simulink model "Modeling"  (R2022b)
settings: Solver=VariableStepAuto  StartTime=0.0  StopTime=2.5  RelTol=1e-3
values from neighbouring files (symbols this model uses):
  b_m = 0.002953    [Modeling_constants.m]
  g = 9.81    [Modeling_constants.m]
  j_m = 0.0221    [Modeling_constants.m]
  j_w = 0.01581762    [Modeling_constants.m]
  K_b = 0.25    [Modeling_constants.m]
  K_m = 0.516    [Modeling_constants.m]
  L_a = 0.0281    [Modeling_constants.m]
  M = 1 / 2    (= 0.5)    [Modeling_constants.m]
  m = 0.5    [Modeling_constants.m]
  r = 0.0325    [Modeling_constants.m]
  R_a = 2.581    [Modeling_constants.m]
  V_i = 450    [Modeling_constants.m]
libraries: slpidlib x2
settings Model: Creator=a7mad  LastModifiedBy=a7mad

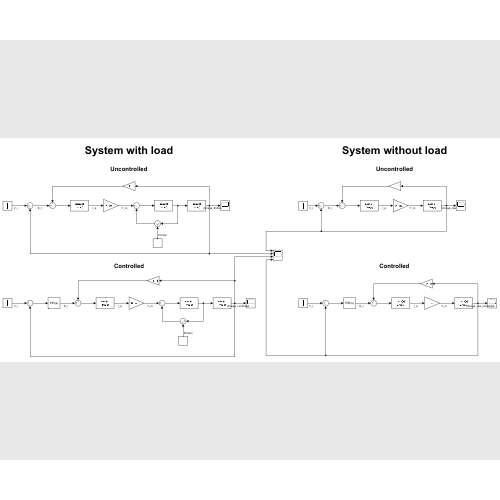
[thumbnail: Simulink's stored preview of the top-level diagram]
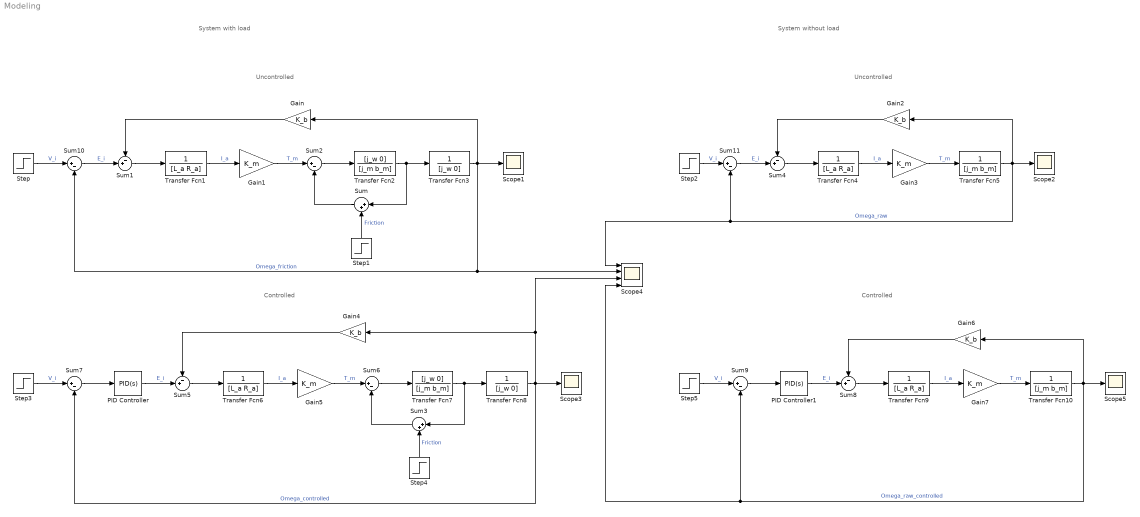
== system Modeling ==
  note: Uncontrolled
  note: Uncontrolled
  note: System with load
  note: System without load
  note: Controlled
  note: Controlled
  Gain{,2,4,6} (4 alike) : Gain  Gain=K_b
  Gain{1,3,5,7} (4 alike) : Gain  Gain=K_m
  PID Controller : slpidlib/PID Controller  Controller=PID  Form=Parallel  TimeDomain=Continuous-time  UseExternalTs=off  SampleTime=-1  IntegratorMethod=Forward Euler  FilterMethod=Forward Euler  ControllerParametersSource=internal  P=9.43501781949502  I=75.7014962747776  UseKiTs=off  D=0.128239684517164  N=5714.13988020802  UseFilter=on  TunerSelectOption=Transfer Function Based (PID Tuner App)  InitialConditionSource=internal  InitialConditionForIntegrator=0  InitialConditionForFilter=0  DifferentiatorICPrevScaledInput=0  ExternalReset=none  TrackingMode=off  Kt=1  LimitOutput=off  SatLimitsSource=internal  UpperSaturationLimit=250  LowerSaturationLimit=0  LinearizeAsGain=off  AntiWindupMode=none  Kb=1  LimitIntegrator=off  UpperIntegratorSaturationLimit=inf  LowerIntegratorSaturationLimit=-inf  POutMin=[]  POutMax=[]  IOutMin=[]  IOutMax=[]  DOutMin=[]  DOutMax=[]  NOutMin=[]  NOutMax=[]  SumOutMin=[]  SumOutMax=[]  SaturationOutMin=[]  SaturationOutMax=[]  PParamMin=[]  PParamMax=[]  IParamMin=[]  IParamMax=[]  DParamMin=[]  DParamMax=[]  NParamMin=[]  NParamMax=[]  KbParamMin=[]  KbParamMax=[]  KtParamMin=[]  KtParamMax=[]  KbOutMin=[]  KbOutMax=[]  KtOutMin=[]  KtOutMax=[]  IntegratorOutMin=[]  IntegratorOutMax=[]  FilterOutMin=[]  FilterOutMax=[]  SumI1OutMin=[]  SumI1OutMax=[]  SumI2OutMin=[]  SumI2OutMax=[]  SumI3OutMin=[]  SumI3OutMax=[]  SumI4OutMin=[]  SumI4OutMax=[]  SumDOutMin=[]  SumDOutMax=[]  DifferentiatorOutMin=[]  DifferentiatorOutMax=[]  FilterDiffOutCoefMin=[]  FilterDiffOutCoefMax=[]  ReciprocalOutMin=[]  ReciprocalOutMax=[]  SumDenOutMin=[]  SumDenOutMax=[]  SumNumOutMin=[]  SumNumOutMax=[]  DivideOutMin=[]  DivideOutMax=[]  UdiffTsProdOutMin=[]  UdiffTsProdOutMax=[]  NTsProdOutMin=[]  NTsProdOutMax=[]  UintegralTsProdOutMin=[]  UintegralTsProdOutMax=[]  UngainTsProdOutMin=[]  UngainTsProdOutMax=[]  ClampingZeroOutDataTypeStr=Inherit: Inherit via back propagation  ClampingZeroOutMin=[]  ClampingZeroOutMax=[]  FilterDenConstantOutDataTypeStr=Inherit: Inherit via back propagation  FilterDenConstantOutMin=[]  FilterDenConstantOutMax=[]  PCopyOutDataTypeStr=Inherit: Inherit via back propagation  PCopyOutMin=[]  PCopyOutMax=[]  NCopyOutDataTypeStr=Inherit: Inherit via back propagation  NCopyOutMin=[]  NCopyOutMax=[]  IntegratorContinuousStateAttributes=''  IntegratorStateMustResolveToSignalObject=off  IntegratorRTWStateStorageClass=Auto  FilterContinuousStateAttributes=''  FilterStateMustResolveToSignalObject=off  FilterRTWStateStorageClass=Auto  ParallelPVariant=InternalParameters  IdealPVariant=Disabled  IVariant=InternalParameters  DVariant=InternalParameters  IntegratorVariant=Continuous  SatVariant=Disabled  AWVariant=Passthrough  PCopyVariant=Disabled  TRVariant=Disabled  FdbkBlocksVariant=Forward  IdealPFdbkVariant=Disabled  SatFdbkVariant=Disabled  DerivativeFilterVariant=ContFilter  NVariant=InternalParameters  NCopyVariant=Disabled  FilterICVariant=InternalICsFilter  IntegratorICVariant=InternalICs  ExternalResetVariant=Disabled  TRSumVariant=Passthrough  SumFdbkVariant=Disabled  SumVariant=Sum_PID  TsampFilterVariant=InternalTs  TsampNgainVariant=Passthrough  TsampIntegralVariant=Passthrough  ExternalSaturationOutDataTypeStr=Inherit: Same as second input
  PID Controller1 : slpidlib/PID Controller  Controller=PID  Form=Parallel  TimeDomain=Continuous-time  UseExternalTs=off  SampleTime=-1  IntegratorMethod=Forward Euler  FilterMethod=Forward Euler  ControllerParametersSource=internal  P=7.32618685889846  I=72.9007980371657  UseKiTs=off  D=0.0926720638683543  N=7618.85317361069  UseFilter=on  TunerSelectOption=Transfer Function Based (PID Tuner App)  InitialConditionSource=internal  InitialConditionForIntegrator=0  InitialConditionForFilter=0  DifferentiatorICPrevScaledInput=0  ExternalReset=none  TrackingMode=off  Kt=1  LimitOutput=off  SatLimitsSource=internal  UpperSaturationLimit=250  LowerSaturationLimit=0  LinearizeAsGain=off  AntiWindupMode=none  Kb=1  LimitIntegrator=off  UpperIntegratorSaturationLimit=inf  LowerIntegratorSaturationLimit=-inf  POutMin=[]  POutMax=[]  IOutMin=[]  IOutMax=[]  DOutMin=[]  DOutMax=[]  NOutMin=[]  NOutMax=[]  SumOutMin=[]  SumOutMax=[]  SaturationOutMin=[]  SaturationOutMax=[]  PParamMin=[]  PParamMax=[]  IParamMin=[]  IParamMax=[]  DParamMin=[]  DParamMax=[]  NParamMin=[]  NParamMax=[]  KbParamMin=[]  KbParamMax=[]  KtParamMin=[]  KtParamMax=[]  KbOutMin=[]  KbOutMax=[]  KtOutMin=[]  KtOutMax=[]  IntegratorOutMin=[]  IntegratorOutMax=[]  FilterOutMin=[]  FilterOutMax=[]  SumI1OutMin=[]  SumI1OutMax=[]  SumI2OutMin=[]  SumI2OutMax=[]  SumI3OutMin=[]  SumI3OutMax=[]  SumI4OutMin=[]  SumI4OutMax=[]  SumDOutMin=[]  SumDOutMax=[]  DifferentiatorOutMin=[]  DifferentiatorOutMax=[]  FilterDiffOutCoefMin=[]  FilterDiffOutCoefMax=[]  ReciprocalOutMin=[]  ReciprocalOutMax=[]  SumDenOutMin=[]  SumDenOutMax=[]  SumNumOutMin=[]  SumNumOutMax=[]  DivideOutMin=[]  DivideOutMax=[]  UdiffTsProdOutMin=[]  UdiffTsProdOutMax=[]  NTsProdOutMin=[]  NTsProdOutMax=[]  UintegralTsProdOutMin=[]  UintegralTsProdOutMax=[]  UngainTsProdOutMin=[]  UngainTsProdOutMax=[]  ClampingZeroOutDataTypeStr=Inherit: Inherit via back propagation  ClampingZeroOutMin=[]  ClampingZeroOutMax=[]  FilterDenConstantOutDataTypeStr=Inherit: Inherit via back propagation  FilterDenConstantOutMin=[]  FilterDenConstantOutMax=[]  PCopyOutDataTypeStr=Inherit: Inherit via back propagation  PCopyOutMin=[]  PCopyOutMax=[]  NCopyOutDataTypeStr=Inherit: Inherit via back propagation  NCopyOutMin=[]  NCopyOutMax=[]  IntegratorContinuousStateAttributes=''  IntegratorStateMustResolveToSignalObject=off  IntegratorRTWStateStorageClass=Auto  FilterContinuousStateAttributes=''  FilterStateMustResolveToSignalObject=off  FilterRTWStateStorageClass=Auto  ParallelPVariant=InternalParameters  IdealPVariant=Disabled  IVariant=InternalParameters  DVariant=InternalParameters  IntegratorVariant=Continuous  SatVariant=Disabled  AWVariant=Passthrough  PCopyVariant=Disabled  TRVariant=Disabled  FdbkBlocksVariant=Forward  IdealPFdbkVariant=Disabled  SatFdbkVariant=Disabled  DerivativeFilterVariant=ContFilter  NVariant=InternalParameters  NCopyVariant=Disabled  FilterICVariant=InternalICsFilter  IntegratorICVariant=InternalICs  ExternalResetVariant=Disabled  TRSumVariant=Passthrough  SumFdbkVariant=Disabled  SumVariant=Sum_PID  TsampFilterVariant=InternalTs  TsampNgainVariant=Passthrough  TsampIntegralVariant=Passthrough  ExternalSaturationOutDataTypeStr=Inherit: Same as second input
  Scope{1..3,5} (4 alike) : Scope
  Scope4 : Scope  NumInputPorts=4
  Step{,2..3,5} (4 alike) : Step  Time=0  After=V_i  SampleTime=0
  Step1 : Step  Time=0  After=M * g * m * r  SampleTime=0
  Step4 : Step  Time=0  After=M * g * m * r  SampleTime=0
  Sum : Sum  Inputs=|++
  Sum{1,4..5,8} (4 alike) : Sum  Inputs=-+|
  Sum{2,6..7,9..11} (6 alike) : Sum  Inputs=|+-
  Sum3 : Sum  Inputs=|++
  Transfer Fcn{1,4,6,9} (4 alike) : TransferFcn  Denominator=[L_a R_a]
  Transfer Fcn10 : TransferFcn  Denominator=[j_m b_m]
  Transfer Fcn2 : TransferFcn  Numerator=[j_w 0]  Denominator=[j_m b_m]
  Transfer Fcn3 : TransferFcn  Denominator=[j_w 0]
  Transfer Fcn5 : TransferFcn  Denominator=[j_m b_m]
  Transfer Fcn7 : TransferFcn  Numerator=[j_w 0]  Denominator=[j_m b_m]
  Transfer Fcn8 : TransferFcn  Denominator=[j_w 0]
  wires:
  Sum1/1 -> Transfer Fcn1/1
  Transfer Fcn1/1 -> Gain1/1  "I_a"
  Gain1/1 -> Sum2/1  "T_m"
  Sum2/1 -> Transfer Fcn2/1
  Transfer Fcn2/1 -> Sum/1, Transfer Fcn3/1
  Gain/1 -> Sum1/1
  Step1/1 -> Sum/2  "Friction"
  Transfer Fcn3/1 -> Sum10/2, Scope4/2, Gain/1, Scope1/1  "Omega_friction"
  Sum/1 -> Sum2/2
  Gain2/1 -> Sum4/1
  Transfer Fcn4/1 -> Gain3/1  "I_a"
  Sum4/1 -> Transfer Fcn4/1
  Gain3/1 -> Transfer Fcn5/1  "T_m"
  Transfer Fcn5/1 -> Sum11/2, Scope4/1, Gain2/1, Scope2/1  "Omega_raw"
  Sum3/1 -> Sum6/2
  Transfer Fcn8/1 -> Scope4/3, Gain4/1, Sum7/2, Scope3/1  "Omega_controlled"
  Step4/1 -> Sum3/2  "Friction"
  Gain4/1 -> Sum5/1
  Transfer Fcn7/1 -> Transfer Fcn8/1, Sum3/1
  Sum6/1 -> Transfer Fcn7/1
  Gain5/1 -> Sum6/1  "T_m"
  Transfer Fcn6/1 -> Gain5/1  "I_a"
  Sum5/1 -> Transfer Fcn6/1
  Step3/1 -> Sum7/1  "V_i"
  Sum7/1 -> PID Controller/1
  PID Controller/1 -> Sum5/2  "E_i"
  Transfer Fcn10/1 -> Scope4/4, Sum9/2, Scope5/1, Gain6/1  "Omega_raw_controlled"
  Gain7/1 -> Transfer Fcn10/1  "T_m"
  Sum8/1 -> Transfer Fcn9/1
  Transfer Fcn9/1 -> Gain7/1  "I_a"
  Gain6/1 -> Sum8/1
  Step5/1 -> Sum9/1  "V_i"
  Sum9/1 -> PID Controller1/1
  PID Controller1/1 -> Sum8/2  "E_i"
  Step2/1 -> Sum11/1  "V_i"
  Sum11/1 -> Sum4/2  "E_i"
  Step/1 -> Sum10/1  "V_i"
  Sum10/1 -> Sum1/2  "E_i"
